simulink model "ModelValidation"  (R2020b)
settings: Solver=ode15s  StartTime=0.0  StopTime=Tsim  RelTol=1e-3
undefined symbols (not defined in the file or in its folder): AA, h0, xv, ygamma1, ygamma2, yk1, yk2
libraries: simulink x4, simulink_extras x4
settings Model: Creator=fabio  LastModifiedBy=fabio
settings DebuggingCC: UnconnectedInputMsg=none  UnconnectedOutputMsg=none  UnconnectedLineMsg=none
settings ModelReferenceCC: EnableRefExpFcnMdlSchedulingChecks=off

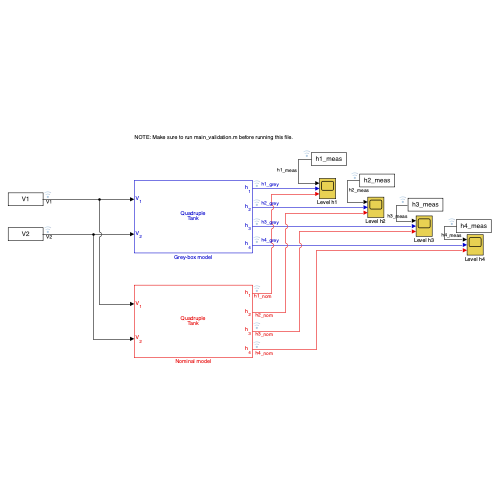
[thumbnail: Simulink's stored preview of the top-level diagram]
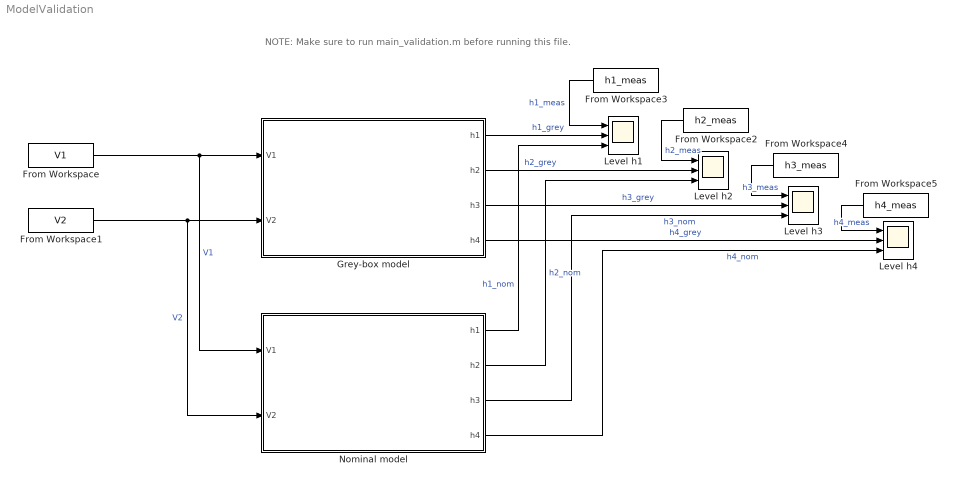
== system ModelValidation ==
  note: NOTE: Make sure to run main_validation.m before running this file.
  From Workspace : FromWorkspace  VariableName=V1  SampleTime=-1  OutputAfterFinalValue=Holding final value
  From Workspace1 : FromWorkspace  VariableName=V2  SampleTime=-1  OutputAfterFinalValue=Holding final value
  From Workspace2 : FromWorkspace  VariableName=h2_meas  SampleTime=-1
  From Workspace3 : FromWorkspace  VariableName=h1_meas  SampleTime=-1
  From Workspace4 : FromWorkspace  VariableName=h3_meas  SampleTime=-1
  From Workspace5 : FromWorkspace  VariableName=h4_meas  SampleTime=-1
  Grey-box model : Subsystem  mask{h_0=h0, A=AA, S=(4.44 / 2)^2 * pi * ones(1, 4), g=981}
      mask prompts: h_0 "Initial level"; A "Outlet section"; S "Tank section"; g "Gravity"
      mask DialogControl h_0 Tooltip: [cm]
      mask DialogControl A Tooltip: [cm^2]
      mask DialogControl S Tooltip: [cm^2]
      mask DialogControl g Tooltip: [cm/s^2]
      mask Display:
      | disp('Quadruple\nTank');
      | port_label('input', 1, 'V_1', 'interpreter', 'tex');
      | port_label('input', 2, 'V_2', 'interpreter', 'tex');
      | port_label('output', 1, 'h_1', 'interpreter', 'tex');
      | port_label('output', 2, 'h_2', 'interpreter', 'tex');
      | port_label('output', 3, 'h_3', 'interpreter', 'tex');
      | port_label('output', 4, 'h_4', 'interpreter', 'tex');
  Level h{1..4} (4 alike) : Scope  NumInputPorts=3
  Nominal model : Subsystem  mask{h_0=h0, A=[0.0792, 0.2425, 0.0792, 0.2425], S=(4.44 / 2)^2 * pi * ones(1, 4), g=981}
      mask prompts: h_0 "Initial level"; A "Outlet section"; S "Tank section"; g "Gravity"
      mask DialogControl h_0 Tooltip: [cm]
      mask DialogControl A Tooltip: [cm^2]
      mask DialogControl S Tooltip: [cm^2]
      mask DialogControl g Tooltip: [cm/s^2]
      mask Display:
      | disp('Quadruple\nTank');
      | port_label('input', 1, 'V_1', 'interpreter', 'tex');
      | port_label('input', 2, 'V_2', 'interpreter', 'tex');
      | port_label('output', 1, 'h_1', 'interpreter', 'tex');
      | port_label('output', 2, 'h_2', 'interpreter', 'tex');
      | port_label('output', 3, 'h_3', 'interpreter', 'tex');
      | port_label('output', 4, 'h_4', 'interpreter', 'tex');
  wires:
  From Workspace/1 -> Nominal model/1(V1), Grey-box model/1(V1)  "V1"
  From Workspace1/1 -> Nominal model/2(V2), Grey-box model/2(V2)  "V2"
  Grey-box model/1(h1) -> Level h1/2  "h1_grey"
  From Workspace3/1 -> Level h1/1  "h1_meas"
  From Workspace2/1 -> Level h2/1  "h2_meas"
  Grey-box model/2(h2) -> Level h2/2  "h2_grey"
  From Workspace4/1 -> Level h3/1  "h3_meas"
  Grey-box model/3(h3) -> Level h3/2  "h3_grey"
  Grey-box model/4(h4) -> Level h4/2  "h4_grey"
  From Workspace5/1 -> Level h4/1  "h4_meas"
  Nominal model/4(h4) -> Level h4/3  "h4_nom"
  Nominal model/3(h3) -> Level h3/3  "h3_nom"
  Nominal model/2(h2) -> Level h2/3  "h2_nom"
  Nominal model/1(h1) -> Level h1/3  "h1_nom"

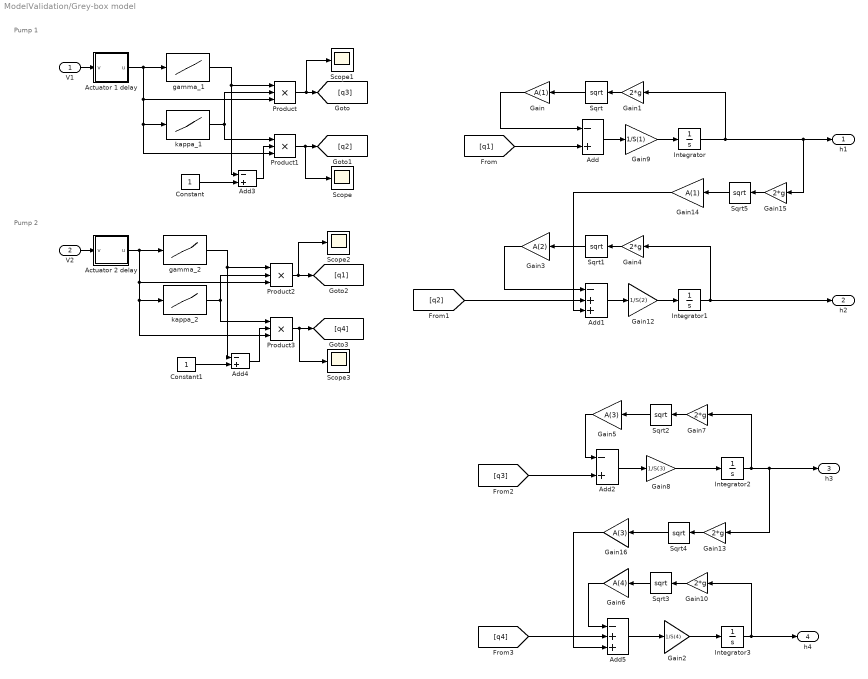
== system ModelValidation/Grey-box model ==
  note: Pump 1
  note: Pump 2
  V1 : Inport
  V2 : Inport  Port=2
  Actuator 1 delay : Subsystem
  Actuator 2 delay : Subsystem
  Add{,2..4} (4 alike) : Sum  Inputs=-+
  Add1 : Sum  Inputs=-++
  Add5 : Sum  Inputs=-++
  Constant : Constant
  Constant1 : Constant
  Gain : Gain  Gain=A(1)
  Gain{1,4,7,10,13,15} (6 alike) : Gain  Gain=2*g
  Gain12 : Gain  Gain=1/S(2)
  Gain14 : Gain  Gain=A(1)
  Gain16 : Gain  Gain=A(3)
  Gain2 : Gain  Gain=1/S(4)
  Gain3 : Gain  Gain=A(2)
  Gain5 : Gain  Gain=A(3)
  Gain6 : Gain  Gain=A(4)
  Gain8 : Gain  Gain=1/S(3)
  Gain9 : Gain  Gain=1/S(1)
  Integrator : Integrator  InitialCondition=h_0(1)  LimitOutput=on  UpperSaturationLimit=30  LowerSaturationLimit=0
  Integrator1 : Integrator  InitialCondition=h_0(2)  LimitOutput=on  UpperSaturationLimit=30  LowerSaturationLimit=0
  Integrator2 : Integrator  InitialCondition=h_0(3)  LimitOutput=on  UpperSaturationLimit=30  LowerSaturationLimit=0
  Integrator3 : Integrator  InitialCondition=h_0(4)  LimitOutput=on  UpperSaturationLimit=30  LowerSaturationLimit=0
  Product{,1..3} (4 alike) : Product  Inputs=3
  Scope{,1..3} (4 alike) : Scope
  Sqrt{,1..5} (6 alike) : Sqrt  SaturateOnIntegerOverflow=on
  gamma_1 : Lookup_n-D  NumberOfTableDimensions=1  BreakpointsForDimension1=xv  Table=ygamma1  ExtrapMethod=Clip  UseLastTableValue=on  InternalRulePriority=Speed  RndMeth=Simplest  InputSameDT=on
  gamma_2 : Lookup_n-D  NumberOfTableDimensions=1  BreakpointsForDimension1=xv  Table=ygamma2  ExtrapMethod=Clip  UseLastTableValue=on  InternalRulePriority=Speed  RndMeth=Simplest  InputSameDT=on
  kappa_1 : Lookup_n-D  NumberOfTableDimensions=1  BreakpointsForDimension1=xv  Table=yk1  ExtrapMethod=Clip  UseLastTableValue=on  InternalRulePriority=Speed  RndMeth=Simplest  InputSameDT=on
  kappa_2 : Lookup_n-D  NumberOfTableDimensions=1  BreakpointsForDimension1=xv  Table=yk2  ExtrapMethod=Clip  UseLastTableValue=on  InternalRulePriority=Speed  RndMeth=Simplest  InputSameDT=on
  h1 : Outport
  h2 : Outport  Port=2
  h3 : Outport  Port=3
  h4 : Outport  Port=4
  wires:
  Integrator/1 -> Gain15/1, h1/1, Gain1/1
  Gain1/1 -> Sqrt/1
  Sqrt/1 -> Gain/1
  Gain/1 -> Add/1
  [q1] -> Add/2
  Add1/1 -> Gain12/1
  Integrator1/1 -> Gain4/1, h2/1
  Gain4/1 -> Sqrt1/1
  Add2/1 -> Gain8/1
  Gain7/1 -> Sqrt2/1
  Sqrt2/1 -> Gain5/1
  Gain6/1 -> Add5/1
  Sqrt3/1 -> Gain6/1
  Gain10/1 -> Sqrt3/1
  Integrator3/1 -> Gain10/1, h4/1
  [q4] -> Add5/2
  Sqrt4/1 -> Gain16/1
  Gain13/1 -> Sqrt4/1
  Integrator2/1 -> Gain7/1, h3/1, Gain13/1
  Sqrt1/1 -> Gain3/1
  Gain3/1 -> Add1/1
  Gain5/1 -> Add2/1
  Gain15/1 -> Sqrt5/1
  Sqrt5/1 -> Gain14/1
  Gain14/1 -> Add1/3
  [q2] -> Add1/2
  [q3] -> Add2/2
  Gain16/1 -> Add5/3
  V1/1 -> Actuator 1 delay/1(v)
  gamma_1/1 -> Add3/1, Product/1
  Constant/1 -> Add3/2
  kappa_1/1 -> Product/2, Product1/1
  Add3/1 -> Product1/2
  Product/1 -> Scope1/1, [q3]
  Product1/1 -> Scope/1, [q2]
  kappa_2/1 -> Product3/1, Product2/2
  Product2/1 -> Scope2/1, [q1]
  Constant1/1 -> Add4/2
  gamma_2/1 -> Add4/1, Product2/1
  Product3/1 -> Scope3/1, [q4]
  Add4/1 -> Product3/2
  V2/1 -> Actuator 2 delay/1(v)
  Gain12/1 -> Integrator1/1
  Add/1 -> Gain9/1
  Gain9/1 -> Integrator/1
  Gain8/1 -> Integrator2/1
  Add5/1 -> Gain2/1
  Gain2/1 -> Integrator3/1
  Actuator 1 delay/1(u) -> gamma_1/1, Product/3, kappa_1/1, Product1/3
  Actuator 2 delay/1(u) -> gamma_2/1, Product2/3, kappa_2/1, Product3/3

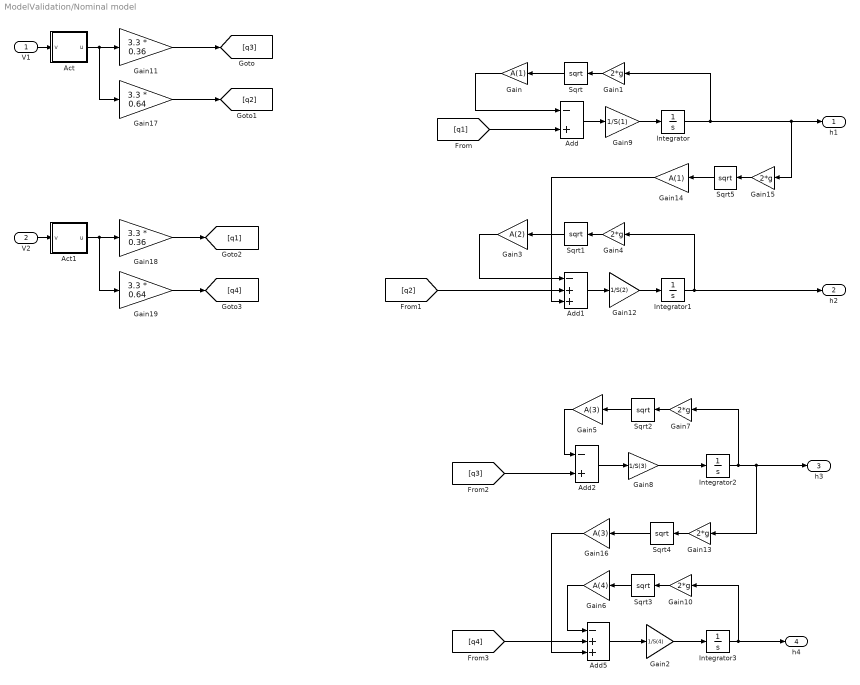
== system ModelValidation/Nominal model ==
  V1 : Inport
  V2 : Inport  Port=2
  Act : Subsystem
  Act1 : Subsystem
  Add : Sum  Inputs=-+
  Add1 : Sum  Inputs=-++
  Add2 : Sum  Inputs=-+
  Add5 : Sum  Inputs=-++
  Gain : Gain  Gain=A(1)
  Gain{1,4,7,10,13,15} (6 alike) : Gain  Gain=2*g
  Gain11 : Gain  Gain=3.3 * 0.36
  Gain12 : Gain  Gain=1/S(2)
  Gain14 : Gain  Gain=A(1)
  Gain16 : Gain  Gain=A(3)
  Gain17 : Gain  Gain=3.3 * 0.64
  Gain18 : Gain  Gain=3.3 * 0.36
  Gain19 : Gain  Gain=3.3 * 0.64
  Gain2 : Gain  Gain=1/S(4)
  Gain3 : Gain  Gain=A(2)
  Gain5 : Gain  Gain=A(3)
  Gain6 : Gain  Gain=A(4)
  Gain8 : Gain  Gain=1/S(3)
  Gain9 : Gain  Gain=1/S(1)
  Integrator : Integrator  InitialCondition=h_0(1)  LimitOutput=on  UpperSaturationLimit=30  LowerSaturationLimit=0
  Integrator1 : Integrator  InitialCondition=h_0(2)  LimitOutput=on  UpperSaturationLimit=30  LowerSaturationLimit=0
  Integrator2 : Integrator  InitialCondition=h_0(3)  LimitOutput=on  UpperSaturationLimit=30  LowerSaturationLimit=0
  Integrator3 : Integrator  InitialCondition=h_0(4)  LimitOutput=on  UpperSaturationLimit=30  LowerSaturationLimit=0
  Sqrt{,1..5} (6 alike) : Sqrt  SaturateOnIntegerOverflow=on
  h1 : Outport
  h2 : Outport  Port=2
  h3 : Outport  Port=3
  h4 : Outport  Port=4
  wires:
  Integrator/1 -> Gain15/1, h1/1, Gain1/1
  Gain1/1 -> Sqrt/1
  Sqrt/1 -> Gain/1
  Gain/1 -> Add/1
  [q1] -> Add/2
  Add1/1 -> Gain12/1
  Integrator1/1 -> Gain4/1, h2/1
  Gain4/1 -> Sqrt1/1
  Add2/1 -> Gain8/1
  Gain7/1 -> Sqrt2/1
  Sqrt2/1 -> Gain5/1
  Gain6/1 -> Add5/1
  Sqrt3/1 -> Gain6/1
  Gain10/1 -> Sqrt3/1
  Integrator3/1 -> Gain10/1, h4/1
  [q4] -> Add5/2
  Sqrt4/1 -> Gain16/1
  Gain13/1 -> Sqrt4/1
  Integrator2/1 -> Gain7/1, h3/1, Gain13/1
  Sqrt1/1 -> Gain3/1
  Gain3/1 -> Add1/1
  Gain5/1 -> Add2/1
  Gain15/1 -> Sqrt5/1
  Sqrt5/1 -> Gain14/1
  Gain14/1 -> Add1/3
  [q2] -> Add1/2
  [q3] -> Add2/2
  Gain16/1 -> Add5/3
  V1/1 -> Act/1(v)
  V2/1 -> Act1/1(v)
  Gain12/1 -> Integrator1/1
  Add/1 -> Gain9/1
  Gain9/1 -> Integrator/1
  Gain8/1 -> Integrator2/1
  Add5/1 -> Gain2/1
  Gain2/1 -> Integrator3/1
  Act/1(u) -> Gain17/1, Gain11/1
  Gain11/1 -> [q3]
  Gain17/1 -> [q2]
  Gain19/1 -> [q4]
  Act1/1(u) -> Gain19/1, Gain18/1
  Gain18/1 -> [q1]

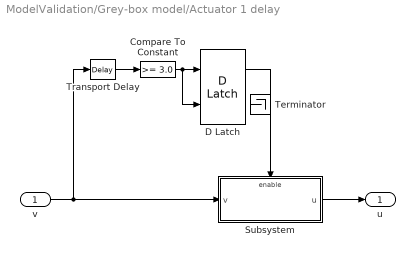
== system ModelValidation/Grey-box model/Actuator 1 delay ==
  v : Inport
  Compare To Constant : simulink/Logic and Bit Operations/Compare To Constant  relop=>=  const=3.0  OutDataTypeStr=boolean
  D Latch : simulink_extras/Flip Flops/D Latch
  Subsystem : Subsystem
  Terminator : Terminator
  Transport Delay : TransportDelay  DelayTime=4
  u : Outport
  wires:
  v/1 -> Transport Delay/1, Subsystem/1(v)
  D Latch/1 -> Subsystem/Enable
  Subsystem/1(u) -> u/1
  Transport Delay/1 -> Compare To Constant/1
  Compare To Constant/1 -> D Latch/2, D Latch/1

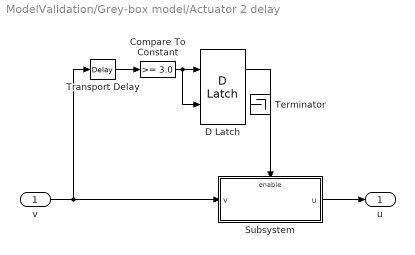
== system ModelValidation/Grey-box model/Actuator 2 delay ==
  v : Inport
  Compare To Constant : simulink/Logic and Bit Operations/Compare To Constant  relop=>=  const=3.0  OutDataTypeStr=boolean
  D Latch : simulink_extras/Flip Flops/D Latch
  Subsystem : Subsystem
  Terminator : Terminator
  Transport Delay : TransportDelay  DelayTime=4
  u : Outport
  wires:
  v/1 -> Transport Delay/1, Subsystem/1(v)
  D Latch/1 -> Subsystem/Enable
  Subsystem/1(u) -> u/1
  Transport Delay/1 -> Compare To Constant/1
  Compare To Constant/1 -> D Latch/2, D Latch/1

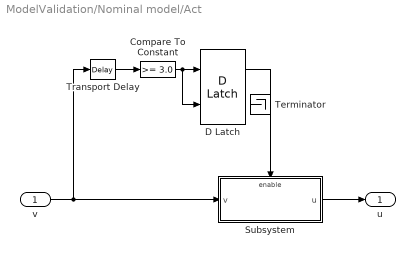
== system ModelValidation/Nominal model/Act ==
  v : Inport
  Compare To Constant : simulink/Logic and Bit Operations/Compare To Constant  relop=>=  const=3.0  OutDataTypeStr=boolean
  D Latch : simulink_extras/Flip Flops/D Latch
  Subsystem : Subsystem
  Terminator : Terminator
  Transport Delay : TransportDelay  DelayTime=4
  u : Outport
  wires:
  v/1 -> Transport Delay/1, Subsystem/1(v)
  D Latch/1 -> Subsystem/Enable
  Subsystem/1(u) -> u/1
  Transport Delay/1 -> Compare To Constant/1
  Compare To Constant/1 -> D Latch/2, D Latch/1

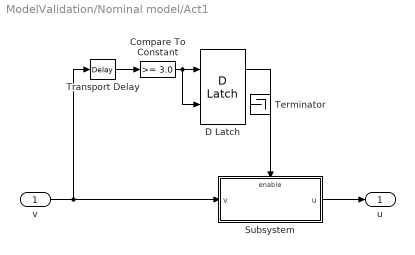
== system ModelValidation/Nominal model/Act1 ==
  v : Inport
  Compare To Constant : simulink/Logic and Bit Operations/Compare To Constant  relop=>=  const=3.0  OutDataTypeStr=boolean
  D Latch : simulink_extras/Flip Flops/D Latch
  Subsystem : Subsystem
  Terminator : Terminator
  Transport Delay : TransportDelay  DelayTime=4
  u : Outport
  wires:
  v/1 -> Transport Delay/1, Subsystem/1(v)
  D Latch/1 -> Subsystem/Enable
  Subsystem/1(u) -> u/1
  Transport Delay/1 -> Compare To Constant/1
  Compare To Constant/1 -> D Latch/2, D Latch/1

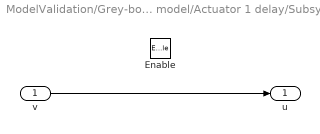
== system ModelValidation/Grey-box model/Actuator 1 delay/Subsystem ==
  v : Inport
  Enable : EnablePort
  u : Outport
  wires:
  v/1 -> u/1

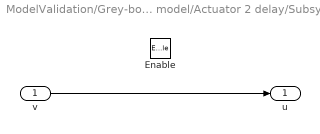
== system ModelValidation/Grey-box model/Actuator 2 delay/Subsystem ==
  v : Inport
  Enable : EnablePort
  u : Outport
  wires:
  v/1 -> u/1

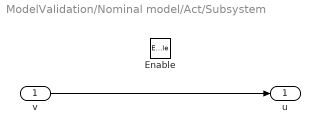
== system ModelValidation/Nominal model/Act/Subsystem ==
  v : Inport
  Enable : EnablePort
  u : Outport
  wires:
  v/1 -> u/1

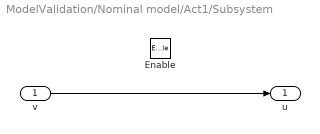
== system ModelValidation/Nominal model/Act1/Subsystem ==
  v : Inport
  Enable : EnablePort
  u : Outport
  wires:
  v/1 -> u/1
